simulink model "question5_model"  (R2021b)
settings: Solver=VariableStepAuto  StartTime=0.0  StopTime=10.0  RelTol=1e-3
settings Model: Creator=stav  LastModifiedBy=stav

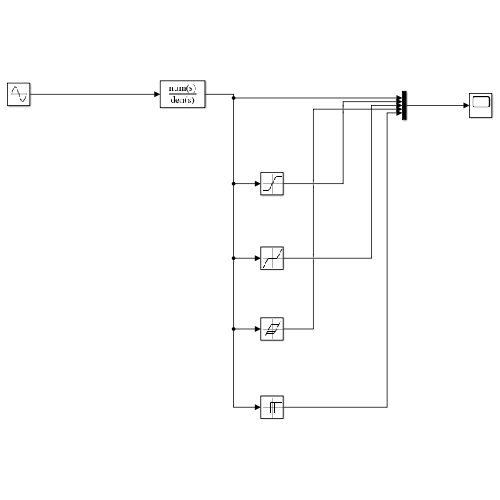
[thumbnail: Simulink's stored preview of the top-level diagram]
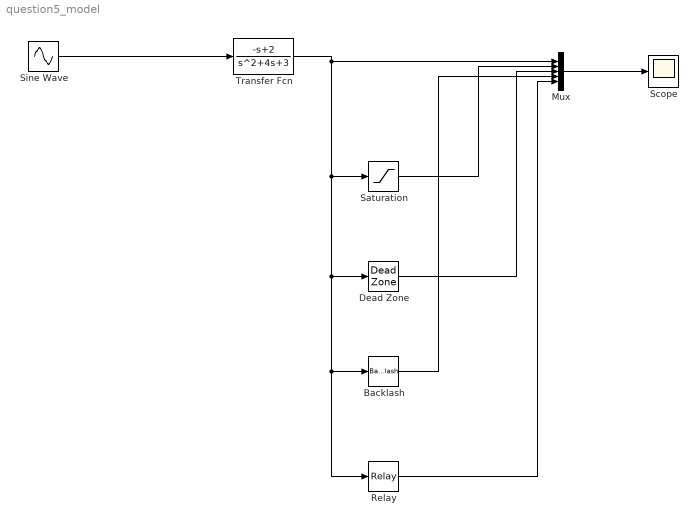
== system question5_model ==
  Backlash : Backlash  BacklashWidth=0.1
  Dead Zone : DeadZone  LowerValue=-0.1  UpperValue=0.1  SaturateOnIntegerOverflow=on
  Mux : Mux  Inputs=5
  Relay : Relay  OnSwitchValue=0.2  OffSwitchValue=-0.2  OnOutputValue=0.2  OffOutputValue=-0.2
  Saturation : Saturate  UpperLimit=0.1  LowerLimit=-0.1
  Scope : Scope
  Sine Wave : Sin  Frequency=5  SampleTime=0
  Transfer Fcn : TransferFcn  Numerator=[-1, 2]  Denominator=[1, 4, 3]
  wires:
  Sine Wave/1 -> Transfer Fcn/1
  Transfer Fcn/1 -> Mux/1, Relay/1, Backlash/1, Dead Zone/1, Saturation/1
  Saturation/1 -> Mux/2
  Dead Zone/1 -> Mux/3
  Mux/1 -> Scope/1
  Relay/1 -> Mux/5
  Backlash/1 -> Mux/4
